simulink model "testemplanner_cs"  (R2020a)
settings: Solver=ode5  StartTime=0.0  StopTime=24  FixedStep=1/1000  RelTol=1e-3
PreLoadFcn:
  | mbxruntime.callbacks.PreLoadFcn(bdroot);
PostLoadFcn:
  | mbxruntime.callbacks.PostLoadFcn(bdroot);
InitFcn:
  | mbxruntime.callbacks.InitFcn(bdroot);
StartFcn:
  | mbxruntime.callbacks.StartFcn(bdroot);
StopFcn:
  | mbxruntime.callbacks.StopFcn(bdroot);
model workspace (MAT data in the model file):
  mbox_table : object (value not decoded)
  model_closed = 0
  sim_status = 0
values from neighbouring files (symbols this model uses):
  c_factor = 43.75    [emplanner_init.m]
  cf = -175016    [emplanner_init.m]
  cr = -130634    [emplanner_init.m]
  global_path_x = [0.057304 1.05668625507 2.05480936558 3.05165624935 4.04722112279 5.04150235808 6.03449985569 7.02621407764 8.01664569183 9.00579544113 9.99366409523 10.9802524329 ... (3001 elements, 3001x1)]    [global_path.mat]
  global_path_y = [8.29 8.29 8.29 8.29 8.29 8.29 8.29 8.29 8.29 8.29 8.29 8.29 ... (3001 elements, 3001x1)]    [global_path.mat]
  KD_PID_distance = 0.0    (= 0)    [emplanner_init.m]
  KD_PID_speed = 0    [emplanner_init.m]
  KI_PID_distance = 0.0    (= 0)    [emplanner_init.m]
  KI_PID_speed = 0    [emplanner_init.m]
  KP_PID_distance = 0.5    [emplanner_init.m]
  KP_PID_speed = 1.8    [emplanner_init.m]
  la = 1.265    [emplanner_init.m]
  lb = 2.947-1.265    (= 1.682)    [emplanner_init.m]
  LQR_K1 = k(:,1)'    [emplanner_init.m]
  LQR_K2 = k(:,2)'    [emplanner_init.m]
  LQR_K3 = k(:,3)'    [emplanner_init.m]
  LQR_K4 = k(:,4)'    [emplanner_init.m]
  m = 2020    [emplanner_init.m]
  rack_displacement = [-39.14 , -37.2 , -35.29 , -33.43 , -31.6 , -29.81 , -28.06 , -26.34 , -24.66 ,      -23.01 , -21.38 , -19.79 , -18.23 , -16.69 , -15.18 , -13.7 , -12.23 , -10.8 , -9.38 , -7.98 ,     -6.61 , -5.25 , -3.91 , -2.59 , -1.29 , 0 , 1.27 , 2.54 , 3.78 , 5.02 , 6.24 , 7.46 , 8.66 ,      9.86 , 11.05 , 12.24 , 13.41 , 14.59 , 15.76 , 16.92 , 18.09 , 19.25 , 20.42 , 21.59 , 22.76 ,      23.93 , 25.11 , 26 ...(+26 chars)    [emplanner_init.m]
  right_wheel_ground = [-70 ,-67.2 , -64.4 , -61.6 , -58.8 , -56 , -53.2 , -50.4 , -47.6 , -44.8 , -42 ,      -39.2 , -36.4 , -33.6 , -30.8 , -28 , -25.2 , -22.4 , -19.6 , -16.8 , -14 , -11.2 , -8.4 , -5.6 ,      -2.8 , 0 , 2.8 , 5.6 , 8.4 , 11.2 , 14 , 16.8 , 19.6 , 22.4 , 25.2 , 28 , 30.8 , 33.6 , 36.4 ,      39.2 , 42 , 44.8 , 47.6 , 50.4 , 53.2 , 56 , 58.8 , 61.6 , 64.4 , 67.2 , 70 ]    [emplanner_init.m]
  vx_break_point = zeros(1,5000)    [emplanner_init.m]
undefined symbols (not defined in the file or in its folder): aubr, DiscIntNeverNeededParam, tablebr, vubr
libraries: PreScanSimulinkLibrary x9, Solver_SF x1, simulink_extras x1
(part 8 of 9)

== matlab function testemplanner_cs/Audi_A8_Sedan_1/decision&planning module/referenceline provider/general fast algorithm to find projection point info1 ==
  data: x_set input; match_point_index_set output; y_set input; path_x input; path_y input; proj_x_set output; proj_y_set output; proj_heading_set output; proj_kappa_set output; path_heading input; path_kappa input
% function [match_point_index_set,proj_x_set,proj_y_set,proj_heading_set,proj_kappa_set] = fcn(x_set,y_set,path_x,path_y,path_heading,path_kappa)
% %该函数是一个通用函数，找到x_set,y_set在path_x,path_y的匹配点的编号，以及投影点在直角坐标系下的(x,y,theta,kappa)
% %最多可以处理128个点
% 
% match_point_index_set = ones(128,1)*nan;
% proj_x_set = ones(128,1)*nan;
% proj_y_set = ones(128,1)*nan;
% proj_heading_set = ones(128,1)*nan;
% proj_kappa_set = ones(128,1)*nan;
% 
% 
% persistent is_first_run;
% persistent init_search_index_set;
% if isempty(is_first_run)
%     is_first_run = 0; 
%     init_search_index_set = ones(128,1)*nan;
%     for i = 1:length(x_set)
%         if isnan(x_set(i))
%             break;
%         else
%             increase_count = 0;
%             min_distance = 1e10;
%             for j = 1:length(path_x)
%                 distance = (x_set(i)-path_x(j))^2 + (y_set(i)-path_y(j))^2;
%                 if (min_distance > distance)
%                     min_distance = distance;
%                     init_search_index_set(i)=j;
%                     increase_count = 0;
%                 else
%                     increase_count = increase_count + 1;
%                 end
%                 if increase_count > 50
%                     break;
%                 end
%             end
%             match_point_index = init_search_index_set(i);
%             match_point_index_set(i) = match_point_index;
%             vector_match_point = [path_x(match_point_index);path_y(match_point_index)];
%             vector_match_point_direction = [cos(path_heading(match_point_index));sin(path_heading(match_point_index))];
%             vector_host_point = [x_set(i);y_set(i)];
%             vector_d = vector_host_point - vector_match_point;
%             vector_err = (vector_d'* vector_match_point_direction) * vector_match_point_direction;
%             vector_proj = vector_err + vector_match_point;
%             proj_x_set(i) = vector_proj(1);
%             proj_y_set(i) = vector_proj(2);
%             proj_heading_set(i) = path_heading(match_point_index) + path_kappa(match_point_index) * (vector_d'* vector_match_point_direction);
%             proj_kappa_set(i) = path_kappa(match_point_index);            
%         end
%     end 
% else
%     min_distance = inf;
%     for i = 1:length(x_set)
%         if isnan(x_set(i))
%             break;
%         else
%             increase_count = 0;
%             start_index = init_search_index_set(i);
%             vector_m_init = [path_x(start_index);path_y(start_index)];
%             vector_direction_init = [cos(path_heading(start_index));sin(path_heading(start_index))];
%             ds = ([x_set(1);y_set(1)]-vector_m_init)'*vector_direction_init;
%             if ds > 0            
%                 for j = start_index:length(path_x)
%                     distance = (x_set(i)-path_x(j))^2 + (y_set(i)-path_y(j))^2;
%                     if (min_distance > distance)
%                         min_distance = distance;
%                         init_search_index_set(i)=j;
%                         increase_count = 0;
%                     else
%                         increase_count = increase_count + 1;
%                     end
%                     if increase_count > 3
%                         break;
%                     end
%                 end
%             else
%                 for j = start_index:-1:1
%                     distance = (x_set(i)-path_x(j))^2 + (y_set(i)-path_y(j))^2;
%                     if (min_distance > distance)
%                         min_distance = distance;
%                         init_search_index_set(i)=j;
%                         increase_count = 0;
%                     else
%                         increase_count = increase_count + 1;
%                     end
%                     if increase_count > 3
%                         break;
%                     end
%                 end
%             end
%             match_point_index = init_search_index_set(i);
%             match_point_index_set(i) = match_point_index;
%             vector_match_point = [path_x(match_point_index);path_y(match_point_index)];
%             vector_match_point_direction = [cos(path_heading(match_point_index));sin(path_heading(match_point_index))];
%             vector_host_point = [x_set(i);y_set(i)];
%             vector_d = vector_host_point - vector_match_point;
%             vector_err = (vector_d'* vector_match_point_direction) * vector_match_point_direction;
%             vector_proj = vector_err + vector_match_point;
%             proj_x_set(i) = vector_proj(1);
%             proj_y_set(i) = vector_proj(2);
%             proj_heading_set(i) = path_heading(match_point_index) + path_kappa(match_point_index) * (vector_d'* vector_match_point_direction);
%             proj_kappa_set(i) = path_kappa(match_point_index);            
%         end
%     end    
% end

function [match_point_index_set,proj_x_set,proj_y_set,proj_heading_set,proj_kappa_set] = fcn(x_set,y_set,path_x,path_y,path_heading,path_kappa)
%该函数是一个通用函数，找到x_set,y_set在path_x,path_y的匹配点的编号，以及投影点在直角坐标系下的(x,y,theta,kappa)
%最多可以处理128个点

match_point_index_set = ones(128,1)*nan;
proj_x_set = ones(128,1)*nan;
proj_y_set = ones(128,1)*nan;
proj_heading_set = ones(128,1)*nan;
proj_kappa_set = ones(128,1)*nan;


persistent is_first_run;
persistent init_search_index_set;
if isempty(is_first_run)
    is_first_run = 0; 
    init_search_index_set = ones(128,1)*nan;
    for i = 1:length(x_set)
        if isnan(x_set(i))
            break;
        else
            increase_count = 0;
            min_distance = 1e10;
            for j = 1:length(path_x)
                distance = (x_set(i)-path_x(j))^2 + (y_set(i)-path_y(j))^2;
                if (min_distance > distance)
                    min_distance = distance;
                    init_search_index_set(i)=j;
                    increase_count = 0;
                else
                    increase_count = increase_count + 1;
                end
                if increase_count > 50
                    break;
                end
            end
            match_point_index = init_search_index_set(i);
            match_point_index_set(i) = match_point_index;
            vector_match_point = [path_x(match_point_index);path_y(match_point_index)];
            vector_match_point_direction = [cos(path_heading(match_point_index));sin(path_heading(match_point_index))];
            vector_host_point = [x_set(i);y_set(i)];
            vector_d = vector_host_point - vector_match_point;
            vector_err = (vector_d'* vector_match_point_direction) * vector_match_point_direction;
            vector_proj = vector_err + vector_match_point;
            proj_x_set(i) = vector_proj(1);
            proj_y_set(i) = vector_proj(2);
            proj_heading_set(i) = path_heading(match_point_index) + path_kappa(match_point_index) * (vector_d'* vector_match_point_direction);
            proj_kappa_set(i) = path_kappa(match_point_index);            
        end
    end 
else
    min_distance = inf;
    for i = 1:length(x_set)
        if isnan(x_set(i))
            break;
        else
            increase_count = 0;
            start_index = init_search_index_set(i);
            vector_m_init = [path_x(start_index);path_y(start_index)];
            vector_direction_init = [cos(path_heading(start_index));sin(path_heading(start_index))];
            ds = ([x_set(1);y_set(1)]-vector_m_init)'*vector_direction_init;

            if ds > 0            
                for j = start_index:length(path_x)
                    distance = (x_set(i)-path_x(j))^2 + (y_set(i)-path_y(j))^2;
                    if (min_distance > distance)
                        min_distance = distance;
                        init_search_index_set(i)=j;
                        increase_count = 0;
                    else
                        increase_count = increase_count + 1;
                    end
                    if increase_count > 3
                        break;
                    end
                end
            else
                for j = start_index:-1:1
                    distance = (x_set(i)-path_x(j))^2 + (y_set(i)-path_y(j))^2;
                    if (min_distance > distance)
                        min_distance = distance;
                        init_search_index_set(i)=j;
                        increase_count = 0;
                    else
                        increase_count = increase_count + 1;
                    end
                    if increase_count > 3
                        break;
                    end
                end
            end
            match_point_index = init_search_index_set(i);
            match_point_index_set(i) = match_point_index;
            vector_match_point = [path_x(match_point_index);path_y(match_point_index)];
            vector_match_point_direction = [cos(path_heading(match_point_index));sin(path_heading(match_point_index))];
            vector_host_point = [x_set(i);y_set(i)];
            vector_d = vector_host_point - vector_match_point;
            vector_err = (vector_d'* vector_match_point_direction) * vector_match_point_direction;
            vector_proj = vector_err + vector_match_point;
            proj_x_set(i) = vector_proj(1);
            proj_y_set(i) = vector_proj(2);
            proj_heading_set(i) = path_heading(match_point_index) + path_kappa(match_point_index) * (vector_d'* vector_match_point_direction);
            proj_kappa_set(i) = path_kappa(match_point_index);            
        end
    end    
end
%    if ds > 0            
%                 for j = start_index:length(path_x)
%                     distance = (x_set(i)-path_x(j))^2 + (y_set(i)-path_y(j))^2;
%                     if (min_distance > distance)
%                         min_distance = distance;
%                         init_search_index_set(i)=j;
%                         increase_count = 0;
%                     else
%                         increase_count = increase_count + 1;
%                     end
%                     if increase_count > 3
%                         break;
%                     end
%                 end
% else
%                 for j = start_index:-1:1
%                     distance = (x_set(i)-path_x(j))^2 + (y_set(i)-path_y(j))^2;
%                     if (min_distance > distance)
%                         min_distance = distance;
%                         init_search_index_set(i)=j;
%                         increase_count = 0;
%                     else
%                         increase_count = increase_count + 1;
%                     end
%                     if increase_count > 3
%                         break;
%                     end
%                 end
%             end
%             match_point_index = init_search_index_set(i);
%             match_point_index_set(i) = match_point_index;
%             vector_match_point = [path_x(match_point_index);path_y(match_point_index)];
%             vector_match_point_direction = [cos(path_heading(match_point_index));sin(path_heading(match_point_index))];
%             vector_host_point = [x_set(i);y_set(i)];
%             vector_d = vector_host_point - vector_match_point;
%             vector_err = (vector_d'* vector_match_point_direction) * vector_match_point_direction;
%             vector_proj = vector_err + vector_match_point;
%             proj_x_set(i) = vector_proj(1);
%             proj_y_set(i) = vector_proj(2);
%             proj_heading_set(i) = path_heading(match_point_index) + path_kappa(match_point_index) * (vector_d'* vector_match_point_direction);
%             proj_kappa_set(i) = path_kappa(match_point_index);            
%         end
%     end    
% end
% 
% 
% 
% 
%

== matlab function testemplanner_cs/Audi_A8_Sedan_1/control module3/control main/lateral control LQR/feedback_control+feedforword_control ==
  data: k input; angle output; err input; forword_angle input
function angle = fcn(k,err,forword_angle)

    angle=-k*err+forword_angle;
end

== matlab function testemplanner_cs/Audi_A8_Sedan_1/control module3/control main/lateral control LQR/predict_module ==
  data: x input; pred_x_ctrl output; y input; phi input; vx input; vy input; phi_dot input; ts input; pred_y_ctrl output; pred_yaw_ctrl output; pred_vx_ctrl output; pred_vy_ctrl output; pred_yaw_dot_ctrl output
function [pred_x_ctrl,pred_y_ctrl,pred_yaw_ctrl,pred_vx_ctrl,pred_vy_ctrl,pred_yaw_dot_ctrl] = fcn(x,y,phi,vx,vy,phi_dot,ts)
    pred_x_ctrl=x+vx*ts*cos(phi)-vy*ts*sin(phi);
    pred_y_ctrl=y+vy*ts*cos(phi)+vx*ts*sin(phi);
    pred_yaw_ctrl=phi;
    pred_vx_ctrl=vx;
    pred_vy_ctrl=vy;
    pred_yaw_dot_ctrl=phi_dot;
end

== matlab function testemplanner_cs/Audi_A8_Sedan_1/control module3/control main/longitudinal control double PID/MATLAB Function1 ==
  data: u input; throttle output; brake output
function [throttle,brake] = fcn(u)
    if u>=0
        throttle=u;
        brake=0;
    else
        throttle=0;
        brake=-u;
    end

== matlab function testemplanner_cs/Audi_A8_Sedan_1/decision&planning module/EM Planner/MATLAB Function1 ==
  data: x_set input; match_point_index_set output; y_set input; frenet_path_x input; frenet_path_y input; frenet_path_heading input; frenet_path_kappa input; proj_x_set output; proj_y_set output; proj_heading_set output; proj_kappa_set output
function [match_point_index_set,proj_x_set, proj_y_set,proj_heading_set,proj_kappa_set] = ...
    fcn(x_set,y_set,frenet_path_x,frenet_path_y,frenet_path_heading,frenet_path_kappa)
%该函数将批量计算x_set，y_set中的xy，在frenet_path下的投影的信息
%输入 x_set,y_set，待投影的点的集合
%x_set,y_set,frenet_path_x,frenet_path_y,frenet_path_heading,frenet_path_kappa
%曲线在直角坐标系下的x，y，heading，kappa
%输出：match_point_index_set 匹配点在frenet_path下的编号的集合(即从全局路径第一个点开始数，第几个点是匹配点)
%     proj_x y heading kappa 投影的x,y,heading,kappa的集合

% 由于事先不知道x_set中到底有多少个点需要投影，因此事先声明一个最大的数量的点作为缓冲
n = 128;
% 并且由于不知道投影点的个数，所以也不知道输出的个数，因此输出也要做缓冲，用nan表示不存在的点
% 输出最多输出128个
% 输出初始化
match_point_index_set = ones(n,1) * nan;
proj_x_set = ones(n,1) * nan;
proj_y_set = ones(n,1) * nan;
proj_heading_set = ones(n,1) * nan;
proj_kappa_set = ones(n,1) * nan;

%找匹配点，需要利用上一个周期的结果作为下一个周期遍历的起点，因此需要声明两个全局变量
persistent is_first_run;
persistent pre_match_point_index_set;
persistent pre_frenet_path_x;
persistent pre_frenet_path_y;
persistent pre_frenet_path_heading;
persistent pre_frenet_path_kappa;
%算法主函数入口

if isempty(is_first_run)
    %该if分支表示函数首次运行
    is_first_run = 0;
    pre_frenet_path_x = frenet_path_x;
    pre_frenet_path_y = frenet_path_y;
    pre_frenet_path_heading = frenet_path_heading;
    pre_frenet_path_kappa = frenet_path_kappa;
    %要记录首次运行计算的匹配点的结果供下个周期运行，先初始化
    pre_match_point_index_set = ones(n,1) * nan;
    %对x_set,y_set的点做遍历，找到他们的匹配点
    for i = 1 : length(x_set)
        if isnan(x_set(i))
            break;
        end
        %首次运行时，没有任何提示，只能从frenet path的第一个点开始找
        start_search_index = 1;
        % 声明increase_count，用于表示在遍历时distance连续增加的个数
        increase_count = 0;
        % 开始遍历
        min_distance = inf;
        for j = start_search_index : length(frenet_path_x)
            distance = (x_set(i) - frenet_path_x(j))^2 + (y_set(i) - frenet_path_y(j))^2;
            if distance < min_distance
                min_distance = distance;
                match_point_index_set(i) = j;
                increase_count = 0;
            else
                increase_count = increase_count + 1;
            end
            %如果distance连续增加50次就不要再遍历了，节省时间
            if increase_count > 50
                break;
            end
        end
        
        %如何通过匹配点计算投影点，请参见《自动驾驶控制算法第七讲》
        %或《自动驾驶决策规划算法》第一章第三节
        
        %取出匹配点的编号
        match_point_index = match_point_index_set(i);
        %取出匹配点的信息
        match_point_x = frenet_path_x(match_point_index);
        match_point_y = frenet_path_y(match_point_index);
        match_point_heading = frenet_path_heading(match_point_index);
        match_point_kappa = frenet_path_kappa(match_point_index);
        %计算匹配点的方向向量与法向量
        vector_match_point = [match_point_x;match_point_y];
        vector_match_point_direction = [cos(match_point_heading);sin(match_point_heading)];
        %声明待投影点的位矢
        vector_r = [x_set(i);y_set(i)];
        
       %通过匹配点计算投影点
       vector_d = vector_r - vector_match_point;
       ds = vector_d' * vector_match_point_direction;
       vector_proj_point = vector_match_point + ds * vector_match_point_direction;
       proj_heading = match_point_heading + match_point_kappa * ds;
       proj_kappa = match_point_kappa;
       %计算结果输出
       proj_x_set(i) = vector_proj_point(1);
       proj_y_set(i) = vector_proj_point(2);
       proj_heading_set(i) = proj_heading;
       proj_kappa_set(i) = proj_kappa;
    end
    %匹配点的计算结果保存，供下一个周期使用
    pre_match_point_index_set = match_point_index_set;
else
    %此if分支表示不是首次运行
    
    %对每个x_set上的点做处理
    for i = 1 : length(x_set)
        %不是首次运行，对于点x_set(i),y_set(i)来说,start_search_index =
        %pre_match_point_index_set(i)
        start_search_index = pre_match_point_index_set(i);%上个周期匹配点的编号作为本周期搜索的起点
        % 声明increase_count，用于表示在遍历时distance连续增加的个数
        %%%%%%%%%
        %对于障碍物检测而言，当感知第一次检测到障碍物时，算法并不是首次运行，此时 
        %pre_match_point_index_set的值是nan，如果还用上一时刻的结果作为本周期搜索的起点
        %必然会出问题，所以要修改
        % 声明increase_count_limit
        increase_count_limit = 5;
        if isnan(start_search_index)
            %没有上个周期的结果，那就不能只检查5次了
            increase_count_limit = 50;
            %搜索起点也要设为1
            start_search_index = 1;
        end
        increase_count = 0;
        % 开始遍历
        %这里多一个步骤，判断遍历的方向
        %计算上个周期匹配点的位矢
        vector_pre_match_point = [pre_frenet_path_x(start_search_index);pre_frenet_path_y(start_search_index)];
        vector_pre_match_point_direction = ...
            [cos(pre_frenet_path_heading(start_search_index));sin(pre_frenet_path_heading(start_search_index))];
        %判断遍历的方向
        flag = ([x_set(i);y_set(i)] - vector_pre_match_point)' * vector_pre_match_point_direction;
        min_distance = inf;
        if flag > 0.001
            for j = start_search_index : length(frenet_path_x)
                distance = (x_set(i) - frenet_path_x(j))^2 + (y_set(i) - frenet_path_y(j))^2;
                if distance < min_distance
                    min_distance = distance;
                    match_point_index_set(i) = j;
                    increase_count = 0;
                else
                    increase_count = increase_count + 1;
                end
                %如果distance连续增加increase_count_limit次就不要再遍历了，节省时间
                if increase_count > increase_count_limit
                    break;
                end
            end
        elseif flag < - 0.001
            for j = start_search_index : -1 : 1
                distance = (x_set(i) - frenet_path_x(j))^2 + (y_set(i) - frenet_path_y(j))^2;
                if distance < min_distance
                    min_distance = distance;
                    match_point_index_set(i) = j;
                    increase_count = 0;
                else
                    increase_count = increase_count + 1;
                end
                %如果distance连续增加increase_count_limit次就不要再遍历了，节省时间
                if increase_count > increase_count_limit
                    break;
                end
            end
        else
            match_point_index_set(i) = start_search_index;
        end
        
        %如何通过匹配点计算投影点，请参见《自动驾驶控制算法第七讲》
        %或《自动驾驶决策规划算法》第一章第三节
        
        %取出匹配点的编号
        match_point_index = match_point_index_set(i);
        %取出匹配点的信息
        match_point_x = frenet_path_x(match_point_index);
        match_point_y = frenet_path_y(match_point_index);
        match_point_heading = frenet_path_heading(match_point_index);
        match_point_kappa = frenet_path_kappa(match_point_index);
        %计算匹配点的方向向量与法向量
        vector_match_point = [match_point_x;match_point_y];
        vector_match_point_direction = [cos(match_point_heading);sin(match_point_heading)];
        %声明待投影点的位矢
        vector_r = [x_set(i);y_set(i)];
        
       %通过匹配点计算投影点
       vector_d = vector_r - vector_match_point;
       ds = vector_d' * vector_match_point_direction;
       vector_proj_point = vector_match_point + ds * vector_match_point_direction;
       proj_heading = match_point_heading + match_point_kappa * ds;
       proj_kappa = match_point_kappa;
       %计算结果输出
       proj_x_set(i) = vector_proj_point(1);
       proj_y_set(i) = vector_proj_point(2);
       proj_heading_set(i) = proj_heading;
       proj_kappa_set(i) = proj_kappa;
  
    end
    %匹配点的计算结果保存，供下一个周期使用
    pre_match_point_index_set = match_point_index_set;
    pre_frenet_path_x = frenet_path_x;
    pre_frenet_path_y = frenet_path_y;
    pre_frenet_path_heading = frenet_path_heading;
    pre_frenet_path_kappa = frenet_path_kappa;
end

== matlab function testemplanner_cs/Audi_A8_Sedan_1/decision&planning module/EM Planner/calc path length and map between point and s ==
  data: trajectory_x input; path_s_end output; trajectory_y input; path_s output
function [path_s_end,path_s] = fcn(trajectory_x,trajectory_y)
% 该函数将计算以trajectory的s 与 x y 的对应关系，可以看作是trajectory index2s
n = length(trajectory_x);
path_s = zeros(n,1);
sum = 0;
for i = 2:length(trajectory_x)
    if isnan(trajectory_x(i))
        break;
    end
    sum = sum + sqrt((trajectory_x(i) - trajectory_x(i-1))^2 + (trajectory_y(i) - trajectory_y(i-1))^2);
    path_s(i) = sum;
end
% 计算出trajectory的长度
if i == n
    path_s_end = path_s(end);
else
    % 因为循环的退出条件为isnan(trajectory_x(i)) 所以 i 所对应的数为 nan 
    path_s_end = path_s(i - 1);
end

== matlab function testemplanner_cs/Audi_A8_Sedan_1/decision&planning module/EM Planner/calc speed planning start condition ==
  data: plan_start_vx input; plan_start_s_dot output; plan_start_vy input; plan_start_ax input; plan_start_ay input; plan_start_heading input; plan_start_s_dot2 output
function [plan_start_s_dot,plan_start_s_dot2] = fcn(plan_start_vx,plan_start_vy,plan_start_ax,plan_start_ay,plan_start_heading)
% 该函数计算速度规划的初始条件
tor = [cos(plan_start_heading);sin(plan_start_heading)];
v_t = tor'*[plan_start_vx;plan_start_vy];
a_t = tor'*[plan_start_ax;plan_start_ay];
plan_start_s_dot = v_t;
plan_start_s_dot2 = a_t;

== matlab function testemplanner_cs/Audi_A8_Sedan_1/decision&planning module/EM Planner/increase st point count ==
  data: s_init input; s output; s_dot_init input; s_dot2_init input; relative_time_init input; s_dot output; s_dot2 output; relative_time output
function [s,s_dot,s_dot2,relative_time] = fcn(s_init,s_dot_init,s_dot2_init,relative_time_init)
%该函数将增密s s_dot s_dot2
% 为什么需要增密，因为控制的执行频率是规划的10倍，轨迹点如果不够密，必然会导致规划效果不好
% 但是若在速度二次规划中点取的太多，会导致二次规划的矩阵规模太大计算太慢
% 所以方法是在二次规划中选取少量的点优化完毕后，在用此函数增密
T = relative_time_init(end);
n = 401;
dt = T/(n-1);
s = zeros(n,1);
s_dot = zeros(n,1);
s_dot2 = zeros(n,1);
relative_time = zeros(n,1);
for i = 1:n
    current_t = (i-1)*dt;
    for j = 1:length(relative_time_init)-1
        if relative_time_init(j) <= current_t && relative_time_init(j+1) > current_t
            break;
        end
    end
    x = current_t - relative_time_init(j);
    s(i) = s_init(j) + s_dot_init(j)*x + (1/3)*s_dot2_init(j)*x^2 + (1/6)*s_dot2_init(j+1)*x^2; 
    s_dot(i) = s_dot_init(j) + 0.5*s_dot2_init(j)*x + 0.5*s_dot2_init(j+1)*x;
    s_dot2(i) = s_dot2_init(j) + (s_dot2_init(j+1) - s_dot2_init(j))*x/(relative_time_init(j+1) - relative_time_init(j));
    relative_time(i) = current_t;
end

== matlab function testemplanner_cs/Audi_A8_Sedan_1/decision&planning module/EM Planner/path and speed merge ==
  data: s input; trajectory_x output; s_dot input; s_dot2 input; relative_time input; current_time input; path_s input; trajectory_x_init input; trajectory_y_init input; trajectory_heading_init input; trajectory_kappa_init input; trajectory_y output; trajectory_heading output; trajectory_kappa output; trajectory_speed output; trajectory_accel output; trajectory_time output
function [trajectory_x,trajectory_y,trajectory_heading,trajectory_kappa,trajectory_speed,trajectory_accel,trajectory_time] = ...
    fcn(s,s_dot,s_dot2,relative_time,current_time,path_s,trajectory_x_init,trajectory_y_init,trajectory_heading_init,trajectory_kappa_init)
% 该函数将合并path和speed
% 由于path 是 60个点，speed 有 401个点，合并后，path和speed有401个点，因此需要做插值
n = 401;
trajectory_x = zeros(n,1);
trajectory_y = zeros(n,1);
trajectory_heading = zeros(n,1);
trajectory_kappa = zeros(n,1);
trajectory_speed = zeros(n,1);

trajectory_accel = zeros(n,1);
index = 1;
% 由于trajectory_x_init中不是所有的值都有效，(有nan) 所以要找到有效值的范围
while ~isnan(trajectory_x_init(index)) 
    index = index + 1;
end
index = index - 1;
trajectory_time = zeros(n,1);
for i = 1:n-1
    %interp1 线性插值
    % 若 x = [1,2] y = [3,4]
    %interp1(x,y,1.5) 会得到3.5
    %interp1 的缺点是 在端点或超过端点的，结果为nan
    % interp1(x,y,2) 不会等于4 而是会等于nan
    % interp1(x,y,6) 也会等于nan，所以在端点处要单独处理
    trajectory_x(i) = interp1(path_s(1:index),trajectory_x_init(1:index),s(i));
    trajectory_y(i) = interp1(path_s(1:index),trajectory_y_init(1:index),s(i));
    trajectory_heading(i) = interp1(path_s(1:index),trajectory_heading_init(1:index),s(i));
    if trajectory_heading(i)==-pi
        trajectory_heading(i)=pi;
    elseif trajectory_heading(i)==(2*pi)||(-2*pi)
        trajectory_heading(i)=0;
    else
    end
    trajectory_kappa(i) = interp1(path_s(1:index),trajectory_kappa_init(1:index),s(i));
    trajectory_time(i) = relative_time(i) + current_time;%速度规划会得到相对时间，转换成绝对时间
    trajectory_speed(i) = s_dot(i);
    trajectory_accel(i) = s_dot2(i);
end
% 端点单独处理
trajectory_x(end) = trajectory_x_init(end);
trajectory_y(end) = trajectory_y_init(end);
trajectory_heading(end) = trajectory_heading_init(end);
trajectory_kappa(end) = trajectory_kappa_init(end);
trajectory_time(end) = relative_time(end) + current_time;
trajectory_speed(end) = s_dot(end);
trajectory_accel(end) = s_dot2(end);

== matlab function testemplanner_cs/Audi_A8_Sedan_1/decision&planning module/EM Planner/Cartesian2Frenet1/MATLAB Function ==
  data: x_set input; s_set output; y_set input; frenet_path_x input; frenet_path_y input; proj_x_set input; proj_y_set input; proj_heading_set input; proj_match_point_index_set input; index2s input; l_set output
function [s_set,l_set] = fcn(x_set,y_set,frenet_path_x,frenet_path_y,...
    proj_x_set,proj_y_set,proj_heading_set,proj_match_point_index_set,index2s)
    %该函数将计算世界坐标系下的x_set，y_set上的点在frenet_path下的坐标s l
    %输入 x_set,y_set 待坐标转换的点
    %     frenet_path_x,frenet_path_y   frenet坐标轴
    %     proj_x,y,heading,kappa,proj_match_point_index 待坐标转换的点的投影点的信息
    %     index2s   frenet_path的index与s的转换表

    % 由于不知道有多少个点需要做坐标转换，所以需要做缓冲
    n = 128;%最多处理128个点
    %输出初始化
    s_set = ones(n,1)*nan;
    l_set = ones(n,1)*nan;
    for i = 1:length(x_set)
        if isnan(x_set(i))
            break;
        end
        %计算s，写个子函数
        s_set(i) = CalcSFromIndex2S(index2s,frenet_path_x,frenet_path_y,proj_x_set(i),proj_y_set(i),...
            proj_match_point_index_set(i));
        n_r = [-sin(proj_heading_set(i));cos(proj_heading_set(i))];
        r_h = [x_set(i);y_set(i)];
        r_r = [proj_x_set(i);proj_y_set(i)];
        l_set(i) = (r_h - r_r)'*n_r;
    end
end

function s = CalcSFromIndex2S(index2s,path_x,path_y,proj_x,proj_y,proj_match_point_index)
  %该函数将计算当指定index2s的映射关系后，计算点proj_x,proj_y的弧长
  vector_1 = [proj_x;proj_y] - [path_x(proj_match_point_index);path_y(proj_match_point_index)];
  %这里要考虑的更全面一些，因为要考虑到proj_match_point_index有可能在path的起点或终点
  if (proj_match_point_index < length(path_x))
      vector_2 = [path_x(proj_match_point_index + 1);path_y(proj_match_point_index + 1)] - ...
          [path_x(proj_match_point_index);path_y(proj_match_point_index)];
  else
      vector_2 = [path_x(proj_match_point_index);path_y(proj_match_point_index)] - ...
          [path_x(proj_match_point_index - 1);path_y(proj_match_point_index - 1)];
  end
  
  if vector_1'*vector_2 > 0
      s = index2s(proj_match_point_index) + sqrt(vector_1'*vector_1);
  else
      s = index2s(proj_match_point_index) - sqrt(vector_1'*vector_1);
  end
  
  
end

== matlab function testemplanner_cs/Audi_A8_Sedan_1/decision&planning module/EM Planner/simple speed qp planning ==
  data: plan_start_s_dot input; s_init output; plan_start_s_dot2 input; s_end input; recommend_T input; s_dot_init output; s_dot2_init output; relative_time_init output
function [s_init,s_dot_init,s_dot2_init,relative_time_init] = fcn(plan_start_s_dot,plan_start_s_dot2,s_end,recommend_T)
%简单速度二次规划
coder.extrinsic("quadprog")
n = 51;
s_init = zeros(n,1);
s_dot_init = zeros(n,1);
s_dot2_init = zeros(n,1);
relative_time_init = zeros(n,1);

Aeq = zeros(3*n,2*n - 2);
beq = zeros(2*n - 2,1);
lb = ones(3*n,1);
ub = lb;
dt = recommend_T/(n-1);
A_sub =[1,0;
        dt,1;
        (1/3)*dt^2,(1/2)*dt;
        -1,0;
        0,-1;
        (1/6)*dt^2,dt/2];
for i = 1:n - 1
    Aeq(3*i-2:3*i+3,2*i-1:2*i) = A_sub;
end

for i = 1:n
   lb(3*i - 2) = -inf;
   lb(3*i - 1) = 0;
   lb(3*i) = -8;
   ub(3*i - 2) = inf;
   ub(3*i - 1) = 50;
   ub(3*i) = 2;
end
lb(1) = 0;
lb(2) = plan_start_s_dot;
lb(3) = plan_start_s_dot2;
ub(1) = lb(1);
ub(2) = lb(2);
ub(3) = lb(3);
lb(3*n - 2) = s_end;
ub(3*n - 2) = s_end;
A3 = zeros(3*n,3*n);
A4 = zeros(3*n,n - 1);
A4_sub =[0;0;1;0;0;-1];
for i = 1:n - 1
   A3(3*i,3*i) = 1;
   A4(3*i-2:3*i+3,i:i) = A4_sub;
end
A3(3*n,3*n) = 1;
H = A3 + 100*(A4*A4');
H = 2*H;
f = zeros(3*n,1);
X = quadprog(H,f,[],[],Aeq',beq,lb,ub);
for i = 1:n
   s_init(i) = X(3*i - 2);
   s_dot_init(i) = X(3*i - 1);
   s_dot2_init(i) = X(3*i);
   relative_time_init(i) = (i - 1)*dt;
end

== matlab function testemplanner_cs/Audi_A8_Sedan_1/decision&planning module/EM_planner1/Cart2Frenet1/CalcSL ==
  data: x_set input; y_set input; referenceline_x input; referenceline_y input; index2s input; plan_start_match_point_index input; plan_start_proj_x input; plan_start_proj_y input; plan_start_proj_heading input; plan_start_proj_kappa input; frenet_s_set output; frenet_l_set output
function [frenet_s_set,frenet_l_set] =fcn(x_set,y_set,referenceline_x,referenceline_y,index2s,plan_start_match_point_index,plan_start_proj_x,plan_start_proj_y,plan_start_proj_heading,plan_start_proj_kappa)
%作用：这是一个通用函数，计算输入的笛卡尔坐标点x,y在自然坐标（frenet）坐标系中的s和l
%输入:要计算的点集的x,y坐标，航向，曲率。他的投影点的x,y坐标，index2s数据，以及参考线数据
%输出：自然坐标系下的s和l
%首先对s和l做一个缓冲
frenet_s_set=ones(128,1)*nan;
frenet_l_set=ones(128,1)*nan;
%开始计算
for i=1:length(x_set)
if isnan(x_set(i))  %遇到空的跳出
    break;
end
%调用相关函数进行s的计算
frenet_s_set(i)=CalcSfromIndex(referenceline_x,referenceline_y,plan_start_proj_x(i),plan_start_proj_y(i),plan_start_match_point_index(i),index2s);

%进行l的计算
%先求自然坐标系的切向量和法向量
%切向量,没用到
%tor=[cos(plan_start_proj_heading(i));sin(plan_start_proj_heading(i))];
%法向量
nor=[-sin(plan_start_proj_heading(i));cos(plan_start_proj_heading(i))];
frenet_l_set(i)=[x_set(i)-plan_start_proj_x(i);y_set(i)-plan_start_proj_y(i)]'*nor;
end

end
function s=CalcSfromIndex(ref_path_x,ref_path_y,match_point_x,match_point_y,match_point_index,index2s)   %使用一个函数来计算index所对应的S值
%%首先判断原点是在匹配点前还是匹配点后，通过向量的内积来进行判断
s_temp =  index2s(match_point_index);
vector1=[match_point_x-ref_path_x(match_point_index);match_point_y-ref_path_y(match_point_index)];
%考虑匹配点在路径终点的情况，不在终点就是匹配点和下一个点作为方向向量，如果是终点则使用匹配点和上一个点作为方向向量
if match_point_index<length(ref_path_x)
    vector2=[ref_path_x(match_point_index+1)-ref_path_x(match_point_index);ref_path_y(match_point_index+1)-ref_path_y(match_point_index)];
else
     vector2=[ref_path_x(match_point_index)-ref_path_x(match_point_index-1);ref_path_y(match_point_index)-ref_path_y(match_point_index-1)];
end
result=vector1'*vector2;    
if result >0 %原点在匹配点后，加上这个距离
    s=s_temp+sqrt(vector1'*vector1);
else        %原点在匹配点前，减去这个距离
    s=s_temp-sqrt(vector1'*vector1);
end
end

== matlab function testemplanner_cs/Audi_A8_Sedan_1/decision&planning module/EM_planner1/Cart2Frenet1/CalcSL2 ==
  data: frenet_l_set input; ax_set input; ay_set input; s_dot_set input; dl_set input; plan_start_proj_heading input; plan_start_proj_kappa input; s_dot2_set output; l_dot2_set output; ddl_set output
function [ s_dot2_set, l_dot2_set,ddl_set]=fcn(frenet_l_set,ax_set,ay_set,s_dot_set,dl_set,plan_start_proj_heading,plan_start_proj_kappa)
%作用：通过之前计算得到的l，s_dot、dl值以及已知的ax，ay值，计算s_dot2,l_dot2,以及ddl
 %首先做一个缓冲
 n=128;
 s_dot2_set=ones(n,1)*nan;
 l_dot2_set=ones(n,1)*nan;
 ddl_set=ones(n,1)*nan;

 for i=1:length(frenet_l_set)
     if isnan(frenet_l_set(i))
         break;
     end
    %先求自然坐标系的切向量和法向量
%切向量
tor=[cos(plan_start_proj_heading(i));sin(plan_start_proj_heading(i))];
%法向量
nor=[-sin(plan_start_proj_heading(i));cos(plan_start_proj_heading(i))];

ah=[ax_set(i);ay_set(i)];
l_dot2_set(i)=ah'*nor- plan_start_proj_kappa(i) * (1 - plan_start_proj_kappa(i) * frenet_l_set(i)) * s_dot_set(i)^2;
s_dot2_set(i)=(1/(1 - plan_start_proj_kappa(i) * frenet_l_set(i)))* (ah' * tor + 2 * plan_start_proj_kappa(i) * dl_set(i) * s_dot_set(i)^2);

if abs(s_dot2_set(i))<1e-6
    ddl_set(i)=0;
else
    ddl_set(i)=(l_dot2_set(i) - dl_set(i)*s_dot2_set(i))/(s_dot_set(i)^2);
 end
end

== matlab function testemplanner_cs/Audi_A8_Sedan_1/decision&planning module/EM_planner1/Cart2Frenet1/Calcs_l_dot_dl ==
  data: frenet_l_set input; vx_set input; vy_set input; plan_start_proj_heading input; plan_start_proj_kappa input; s_dot_set output; l_dot_set output; dl_set output
function [ s_dot_set, l_dot_set,dl_set]=fcn(frenet_l_set,vx_set,vy_set,plan_start_proj_heading,plan_start_proj_kappa)
%作用：通过之前计算得到的s和l值以及计算的速度值，计算s_dot,l_dot,以及dl
 %首先做一个缓冲
 n=128;
 s_dot_set=ones(n,1)*nan;
 l_dot_set=ones(n,1)*nan;
 dl_set=ones(n,1)*nan;

 for i=1:length(frenet_l_set)
     if isnan(frenet_l_set(i))
         break;
     end
    %先求自然坐标系的切向量和法向量
%切向量
tor=[cos(plan_start_proj_heading(i));sin(plan_start_proj_heading(i))];
%法向量
nor=[-sin(plan_start_proj_heading(i));cos(plan_start_proj_heading(i))];

vh=[vx_set(i);vy_set(i)];
l_dot_set(i)=vh'*nor;
s_dot_set(i)=vh'*tor/(1-plan_start_proj_kappa(i)*frenet_l_set(i));

if abs(s_dot_set(i))<1e-6
    dl_set(i)=0;
else
    dl_set(i)=l_dot_set(i)/s_dot_set(i);
 end
end

== matlab function testemplanner_cs/Audi_A8_Sedan_1/decision&planning module/EM_planner1/Cartesian2Frenet/MATLAB Function ==
  data: x_set input; s_set output; y_set input; frenet_path_x input; frenet_path_y input; proj_x_set input; proj_y_set input; proj_heading_set input; proj_match_point_index_set input; index2s input; l_set output
function [s_set,l_set] = fcn(x_set,y_set,frenet_path_x,frenet_path_y,...
    proj_x_set,proj_y_set,proj_heading_set,proj_match_point_index_set,index2s)
    %该函数将计算世界坐标系下的x_set，y_set上的点在frenet_path下的坐标s l
    %输入 x_set,y_set 待坐标转换的点
    %     frenet_path_x,frenet_path_y   frenet坐标轴
    %     proj_x,y,heading,kappa,proj_match_point_index 待坐标转换的点的投影点的信息
    %     index2s   frenet_path的index与s的转换表

    % 由于不知道有多少个点需要做坐标转换，所以需要做缓冲
    n = 128;%最多处理128个点
    %输出初始化
    s_set = ones(n,1)*nan;
    l_set = ones(n,1)*nan;
    for i = 1:length(x_set)
        if isnan(x_set(i))
            break;
        end
        %计算s，写个子函数
        s_set(i) = CalcSFromIndex2S(index2s,frenet_path_x,frenet_path_y,proj_x_set(i),proj_y_set(i),...
            proj_match_point_index_set(i));
        n_r = [-sin(proj_heading_set(i));cos(proj_heading_set(i))];
        r_h = [x_set(i);y_set(i)];
        r_r = [proj_x_set(i);proj_y_set(i)];
        l_set(i) = (r_h - r_r)'*n_r;
    end
end

function s = CalcSFromIndex2S(index2s,path_x,path_y,proj_x,proj_y,proj_match_point_index)
  %该函数将计算当指定index2s的映射关系后，计算点proj_x,proj_y的弧长
  vector_1 = [proj_x;proj_y] - [path_x(proj_match_point_index);path_y(proj_match_point_index)];
  %这里要考虑的更全面一些，因为要考虑到proj_match_point_index有可能在path的起点或终点
  if (proj_match_point_index < length(path_x))
      vector_2 = [path_x(proj_match_point_index + 1);path_y(proj_match_point_index + 1)] - ...
          [path_x(proj_match_point_index);path_y(proj_match_point_index)];
  else
      vector_2 = [path_x(proj_match_point_index);path_y(proj_match_point_index)] - ...
          [path_x(proj_match_point_index - 1);path_y(proj_match_point_index - 1)];
  end
  
  if vector_1'*vector_2 > 0
      s = index2s(proj_match_point_index) + sqrt(vector_1'*vector_1);
  else
      s = index2s(proj_match_point_index) - sqrt(vector_1'*vector_1);
  end
  
  
end

== matlab function testemplanner_cs/Audi_A8_Sedan_1/decision&planning module/EM_planner1/Cartesian2Frenet/MATLAB Function1 ==
  data: l_set input; s_dot_set output; vx_set input; vy_set input; proj_heading_set input; proj_kappa_set input; l_dot_set output; dl_set output
function [s_dot_set,l_dot_set,dl_set] = fcn(l_set,vx_set,vy_set,proj_heading_set,proj_kappa_set)
%该函数将计算frenet坐标系下的s_dot, l_dot, dl/ds
n = 128;
% 输出初始化
s_dot_set = ones(n,1)*nan;
l_dot_set = ones(n,1)*nan;
dl_set = ones(n,1)*nan;

for i = 1 : length(l_set)
    if isnan(l_set(i))
        break;
    end
    v_h = [vx_set(i);vy_set(i)];
    n_r = [-sin(proj_heading_set(i));cos(proj_heading_set(i))];
    t_r = [cos(proj_heading_set(i));sin(proj_heading_set(i))];
    l_dot_set(i) = v_h'*n_r;
    s_dot_set(i) = v_h'*t_r/(1 - proj_kappa_set(i)*l_set(i));
    %%%向量法做cartesian与frenet的转换要更简单，但是也有缺点，向量法必须依赖速度加速度
    %l' = l_dot/s_dot 但是如果s_dot = 0 此方法就失效了
    if abs(s_dot_set(i)) < 1e-6
        dl_set(i) = 0;
    else
        dl_set(i) = l_dot_set(i)/s_dot_set(i);
    end
end

== matlab function testemplanner_cs/Audi_A8_Sedan_1/decision&planning module/EM_planner1/Cartesian2Frenet/MATLAB Function2 ==
  data: ax_set input; s_dot2_set output; ay_set input; proj_heading_set input; proj_kappa_set input; l_set input; s_dot_set input; dl_set input; l_dot2_set output; ddl_set output
function [s_dot2_set,l_dot2_set,ddl_set] = fcn(ax_set,ay_set,proj_heading_set,proj_kappa_set,l_set,s_dot_set,dl_set)
%由于不知道有多少个点需要做坐标转换，设一个最大值做缓冲
n = 128;
% 输出初始化
s_dot2_set = ones(n,1)*nan;
l_dot2_set = ones(n,1)*nan;
ddl_set = ones(n,1)*nan;

for i = 1:length(l_set)
    if isnan(l_set(i))
       break;
    end
    a_h = [ax_set(i);ay_set(i)];
    n_r = [-sin(proj_heading_set(i));cos(proj_heading_set(i))];
    t_r = [cos(proj_heading_set(i));sin(proj_heading_set(i))];
    %近似认为dkr/ds 为0 简化计算
    l_dot2_set(i) = a_h'*n_r - proj_kappa_set(i) * (1 - proj_kappa_set(i) * l_set(i)) * s_dot_set(i)^2;
    s_dot2_set(i) = (1/(1 - proj_kappa_set(i) * l_set(i)))* (a_h' * t_r + 2 * proj_kappa_set(i) * dl_set(i) * s_dot_set(i)^2);
    % 要考虑加速度为0的情况
    if (s_dot2_set(i) < 1e-6)
        ddl_set(i) = 0;
    else
        ddl_set(i) = (l_dot2_set(i) - dl_set(i)*s_dot2_set(i))/(s_dot_set(i)^2);
    end
end

== matlab function testemplanner_cs/Audi_A8_Sedan_1/decision&planning module/EM_planner1/DP node generate ==
  data: dp_path_s_init input; dp_path_s_final output; dp_path_l_init input; plan_start_s input; plan_start_l input; plan_start_dl input; plan_start_ddl input; dp_path_l_final output; dp_path_dl_final output; dp_path_ddl_final output
function [dp_path_s_final,dp_path_l_final,dp_path_dl_final,dp_path_ddl_final] = fcn(dp_path_s_init,dp_path_l_init,plan_start_s,plan_start_l,plan_start_dl,plan_start_ddl)
%%作用：对DP求得的路径进行路径点加密
%%输入：dp求得的点s，l参数，规划起点的s，l，dl，ddl参数
%%输出：加密后的路径点的s，l，dl，ddl参数
%每隔1m取一个点
ds=1;
%初始化输出数组
dp_path_s_final=ones(60,1)*nan;
dp_path_l_final=ones(60,1)*nan;
dp_path_dl_final=ones(60,1)*nan;
dp_path_ddl_final=ones(60,1)*nan;

%初始化过程变量
cur_node_s=0;
l_temp=[];
dl_temp=[];
ddl_temp=[];
%初始化路径起点
start_s=plan_start_s;
start_l=plan_start_l;
start_dl=plan_start_dl;
start_ddl=plan_start_ddl;
%遍历整个输入的s集合，进行节点加密
for i=1:length(dp_path_s_init)
    if dp_path_s_init==-1
        break;
    end
    end_s=dp_path_s_init(i);
    end_l=dp_path_l_init(i);
    end_dl=0;
    end_ddl=0;
    coffee=Calccoffee(start_s,start_l,start_dl,start_ddl,end_s,end_l,end_dl,end_ddl);
    for j=1:10000
        if(start_s+ds*(j-1))<end_s
            cur_node_s=start_s+ds*(j-1);
            l_cur=coffee(1)*(cur_node_s)^5+coffee(2)*(cur_node_s)^4+coffee(3)*(cur_node_s)^3+coffee(4)*(cur_node_s)^2+coffee(5)*(cur_node_s)+coffee(6);
            dl_cur=5*coffee(1)*(cur_node_s)^4+4*coffee(2)*(cur_node_s)^3+3*coffee(3)*(cur_node_s)^2+2*coffee(4)*(cur_node_s)+coffee(5);
            ddl_cur=20*coffee(1)*(cur_node_s)^3+12*coffee(2)*(cur_node_s)^2+6*coffee(3)*(cur_node_s)+2*coffee(4);
            l_temp=[l_temp,l_cur];
            dl_temp=[dl_temp,dl_cur];
            ddl_temp=[ddl_temp,ddl_cur];
            
        else
            break;
        end
    end
      start_s=end_s;
      start_l=end_l;
      start_dl=end_dl;
      start_ddl=end_ddl;
end

for k=1:length(l_temp)
    if k==61
        break;
    else
        dp_path_s_final(k)=plan_start_s+ds*(k-1);
        dp_path_l_final(k)=l_temp(k);
        dp_path_dl_final(k)=dl_temp(k);
        dp_path_ddl_final(k)=ddl_temp(k);
    end
end

end

function coffee=Calccoffee(start_s,start_l,start_dl,start_ddl,end_s,end_l,end_dl,end_ddl)
  %作用：计算五次多项式系数
  %输入：起点和终点的s,l,dl,ddl共6个值
  %输出：六个权重系数
    start_s2=start_s*start_s;
    start_s3=start_s2*start_s;
    start_s4=start_s3*start_s;
    start_s5=start_s4*start_s;
    end_s2=end_s*end_s;
    end_s3=end_s2*end_s;
    end_s4=end_s3*end_s;
    end_s5=end_s4*end_s;
    A=[1,start_s,start_s2,start_s3,start_s4,start_s5;
       0,1,2*start_s,3*start_s2,4*start_s3,5*start_s4;
       0,0,2,6*start_s,12*start_s2,20*start_s3;
       1,end_s,end_s2,end_s3,end_s4,end_s5;
       0,1,2*end_s,3*end_s2,4*end_s3,5*end_s4;
        0,0,2,6*end_s,12*end_s2,20*end_s3;];
    B=[start_l;start_dl;start_ddl;end_l;end_dl;end_ddl];
    coffee=A\B;
end

== matlab function testemplanner_cs/Audi_A8_Sedan_1/decision&planning module/EM_planner1/DP node generate1 ==
  data: dp_path_s_init input; dp_path_s_final output; dp_path_l_init input; plan_start_s input; plan_start_l input; plan_start_dl input; plan_start_ddl input; dp_path_l_final output; dp_path_dl_final output; dp_path_ddl_final output
function [dp_path_s_final,dp_path_l_final,dp_path_dl_final,dp_path_ddl_final] = fcn(dp_path_s_init,dp_path_l_init,plan_start_s,plan_start_l,plan_start_dl,plan_start_ddl)
%%作用：对DP求得的路径进行路径点加密
%%输入：dp求得的点s，l参数，规划起点的s，l，dl，ddl参数
%%输出：加密后的路径点的s，l，dl，ddl参数
%每隔1m取一个点
ds=1;
%初始化输出数组
dp_path_s_final=ones(60,1)*nan;
dp_path_l_final=ones(60,1)*nan;
dp_path_dl_final=ones(60,1)*nan;
dp_path_ddl_final=ones(60,1)*nan;

%初始化过程变量
cur_node_s=0;
l_temp=[];
dl_temp=[];
ddl_temp=[];
%初始化路径起点
start_s=plan_start_s;
start_l=plan_start_l;
start_dl=plan_start_dl;
start_ddl=plan_start_ddl;
%遍历整个输入的s集合，进行节点加密
for i=1:length(dp_path_s_init)
    if dp_path_s_init==-1
        break;
    end
    end_s=dp_path_s_init(i);
    end_l=dp_path_l_init(i);
    end_dl=0;
    end_ddl=0;
    coffee=Calccoffee(start_s,start_l,start_dl,start_ddl,end_s,end_l,end_dl,end_ddl);
    for j=1:10000
        if(start_s+ds*(j-1))<end_s
            cur_node_s=start_s+ds*(j-1);
            l_cur=coffee(1)*(cur_node_s)^5+coffee(2)*(cur_node_s)^4+coffee(3)*(cur_node_s)^3+coffee(4)*(cur_node_s)^2+coffee(5)*(cur_node_s)+coffee(6);
            dl_cur=5*coffee(1)*(cur_node_s)^4+4*coffee(2)*(cur_node_s)^3+3*coffee(3)*(cur_node_s)^2+2*coffee(4)*(cur_node_s)+coffee(5);
            ddl_cur=20*coffee(1)*(cur_node_s)^3+12*coffee(2)*(cur_node_s)^2+6*coffee(3)*(cur_node_s)+2*coffee(4);
            l_temp=[l_temp,l_cur];
            dl_temp=[dl_temp,dl_cur];
            ddl_temp=[ddl_temp,ddl_cur];
            
        else
            break;
        end
    end
      start_s=end_s;
      start_l=end_l;
      start_dl=end_dl;
      start_ddl=end_ddl;
end

for k=1:length(l_temp)
    if k==61
        break;
    else
        dp_path_s_final(k)=plan_start_s+ds*(k-1);
        dp_path_l_final(k)=l_temp(k);
        dp_path_dl_final(k)=dl_temp(k);
        dp_path_ddl_final(k)=ddl_temp(k);
    end
end

end

function coffee=Calccoffee(start_s,start_l,start_dl,start_ddl,end_s,end_l,end_dl,end_ddl)
  %作用：计算五次多项式系数
  %输入：起点和终点的s,l,dl,ddl共6个值
  %输出：六个权重系数
    start_s2=start_s*start_s;
    start_s3=start_s2*start_s;
    start_s4=start_s3*start_s;
    start_s5=start_s4*start_s;
    end_s2=end_s*end_s;
    end_s3=end_s2*end_s;
    end_s4=end_s3*end_s;
    end_s5=end_s4*end_s;
    A=[1,start_s,start_s2,start_s3,start_s4,start_s5;
       0,1,2*start_s,3*start_s2,4*start_s3,5*start_s4;
       0,0,2,6*start_s,12*start_s2,20*start_s3;
       1,end_s,end_s2,end_s3,end_s4,end_s5;
       0,1,2*end_s,3*end_s2,4*end_s3,5*end_s4;
        0,0,2,6*end_s,12*end_s2,20*end_s3;];
    B=[start_l;start_dl;start_ddl;end_l;end_dl;end_ddl];
    coffee=A\B;
end
